simulink model "AccPed"  (R2018a)
settings: configuration reference "cs_ert" (kept outside this file)
settings Model: DataDictionary=AccPed.sldd  Creator=zhoutinglin  LastModifiedBy=zhoutinglin

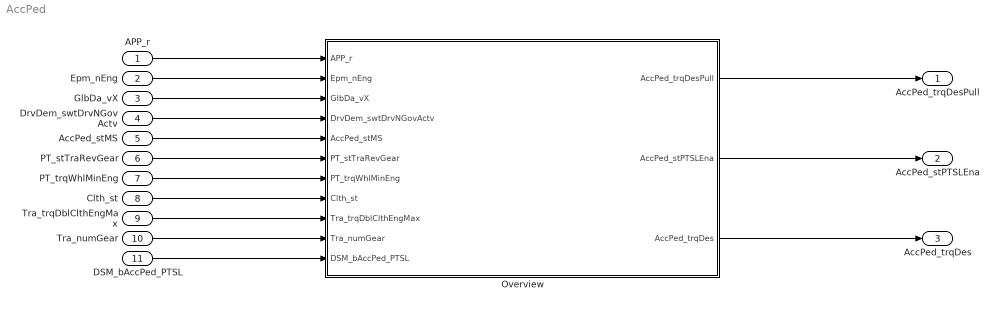
== system AccPed ==
  APP_r : Inport
  Epm_nEng : Inport  Port=2
  GlbDa_vX : Inport  Port=3
  DrvDem_swtDrvNGovActv : Inport  Port=4
  AccPed_stMS : Inport  Port=5
  PT_stTraRevGear : Inport  Port=6
  PT_trqWhlMinEng : Inport  Port=7
  Clth_st : Inport  Port=8
  Tra_trqDblClthEngMax : Inport  Port=9
  Tra_numGear : Inport  Port=10
  DSM_bAccPed_PTSL : Inport  Port=11
  Overview : Subsystem
  AccPed_trqDesPull : Outport
  AccPed_stPTSLEna : Outport  Port=2
  AccPed_trqDes : Outport  Port=3
  wires:
  APP_r/1 -> Overview/1(APP_r)
  Epm_nEng/1 -> Overview/2(Epm_nEng)
  GlbDa_vX/1 -> Overview/3(GlbDa_vX)
  DrvDem_swtDrvNGovActv/1 -> Overview/4(DrvDem_swtDrvNGovActv)
  AccPed_stMS/1 -> Overview/5(AccPed_stMS)
  PT_stTraRevGear/1 -> Overview/6(PT_stTraRevGear)
  PT_trqWhlMinEng/1 -> Overview/7(PT_trqWhlMinEng)
  Clth_st/1 -> Overview/8(Clth_st)
  Tra_trqDblClthEngMax/1 -> Overview/9(Tra_trqDblClthEngMax)
  Tra_numGear/1 -> Overview/10(Tra_numGear)
  DSM_bAccPed_PTSL/1 -> Overview/11(DSM_bAccPed_PTSL)
  Overview/1(AccPed_trqDesPull) -> AccPed_trqDesPull/1
  Overview/2(AccPed_stPTSLEna) -> AccPed_stPTSLEna/1
  Overview/3(AccPed_trqDes) -> AccPed_trqDes/1

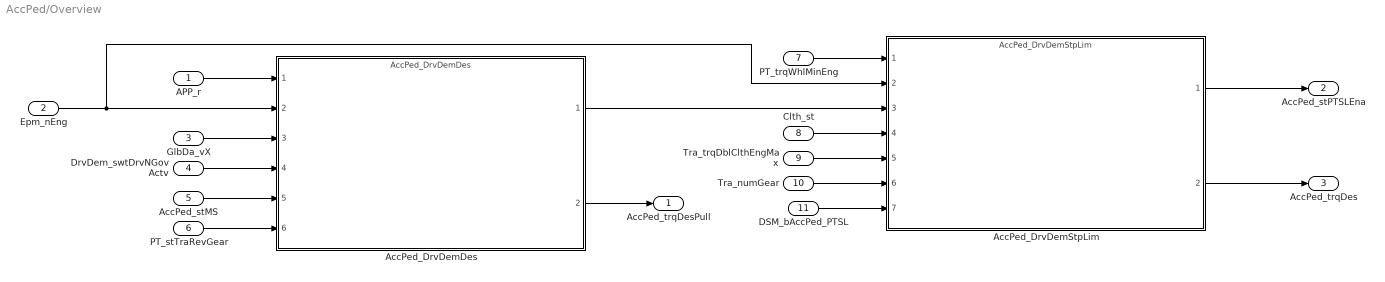
== system AccPed/Overview ==
  APP_r : Inport
  Epm_nEng : Inport  Port=2
  GlbDa_vX : Inport  Port=3
  DrvDem_swtDrvNGovActv : Inport  Port=4
  AccPed_stMS : Inport  Port=5
  PT_stTraRevGear : Inport  Port=6
  PT_trqWhlMinEng : Inport  Port=7
  Clth_st : Inport  Port=8
  Tra_trqDblClthEngMax : Inport  Port=9
  Tra_numGear : Inport  Port=10
  DSM_bAccPed_PTSL : Inport  Port=11
  AccPed_DrvDemDes : ModelReference  ModelNameDialog=AccPed_DrvDemDes  SimulationMode=Normal  ModelReferenceVersion=1.50
  AccPed_DrvDemStpLim : ModelReference  ModelNameDialog=AccPed_DrvDemStpLim  SimulationMode=Normal  ModelReferenceVersion=1.52
  AccPed_trqDesPull : Outport
  AccPed_stPTSLEna : Outport  Port=2
  AccPed_trqDes : Outport  Port=3
  wires:
  AccPed_DrvDemDes/1 -> AccPed_DrvDemStpLim/3
  APP_r/1 -> AccPed_DrvDemDes/1
  Epm_nEng/1 -> AccPed_DrvDemStpLim/2, AccPed_DrvDemDes/2
  GlbDa_vX/1 -> AccPed_DrvDemDes/3
  DrvDem_swtDrvNGovActv/1 -> AccPed_DrvDemDes/4
  AccPed_stMS/1 -> AccPed_DrvDemDes/5
  PT_stTraRevGear/1 -> AccPed_DrvDemDes/6
  AccPed_DrvDemDes/2 -> AccPed_trqDesPull/1
  PT_trqWhlMinEng/1 -> AccPed_DrvDemStpLim/1
  Clth_st/1 -> AccPed_DrvDemStpLim/4
  Tra_trqDblClthEngMax/1 -> AccPed_DrvDemStpLim/5
  Tra_numGear/1 -> AccPed_DrvDemStpLim/6
  DSM_bAccPed_PTSL/1 -> AccPed_DrvDemStpLim/7
  AccPed_DrvDemStpLim/1 -> AccPed_stPTSLEna/1
  AccPed_DrvDemStpLim/2 -> AccPed_trqDes/1
